simulink model "Sim_LQG_LTR_pheno"  (R2015a)
settings: Solver=ode45  StartTime=0.0  StopTime=t_run  RelTol=1e-3
values from neighbouring files (symbols this model uses):
  Cd = SYSd.c    [LQG_LTR_fen.m]    (also in LQG_LTR_ident.m; LQG_LTR_pheno.m)
  Dd = SYSd.d    [LQG_LTR_fen.m]    (also in LQG_LTR_ident.m; LQG_LTR_pheno.m)
  Gamma = SYSd.b    [LQG_LTR_fen.m]    (also in LQG_LTR_ident.m; LQG_LTR_pheno.m)
  hinicial = [9 7 0 0]    [LQG_LTR_fen.m]    (also in LQG_LTR_ident.m; LQG_LTR_pheno.m; Model.m = [hi1 hi2 0 0])
  Kf = minreal(ss(Kc,'minimal'),1e-4)    [LQG_LTR_fen.m]    (also in LQG_LTR_ident.m; LQG_LTR_pheno.m)
  Phi = SYSd.a    [LQG_LTR_fen.m]    (also in LQG_LTR_ident.m; LQG_LTR_pheno.m)
  Ts = 0.1    [LQG_LTR_fen.m]    (also in LQG_LTR_ident.m; LQG_LTR_pheno.m)
settings Model: Creator=pcosta  LastModifiedBy=lca

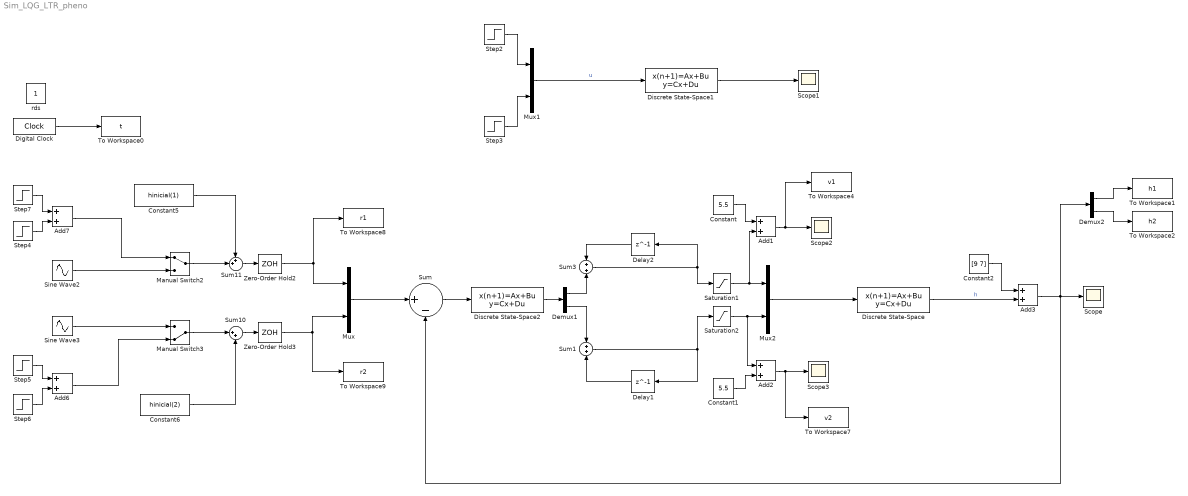
== system Sim_LQG_LTR_pheno ==
  Add{1..3,6..7} (5 alike) : Sum
  Constant : Constant  Value=5.5
  Constant1 : Constant  Value=5.5
  Constant2 : Constant  Value=[9 7]
  Constant5 : Constant  Value=hinicial(1)  SampleTime=Ts
  Constant6 : Constant  Value=hinicial(2)  SampleTime=Ts
  Delay1 : Delay  DelayLength=1  InitialCondition=0  SampleTime=Ts
  Delay2 : Delay  DelayLength=1  InitialCondition=0  SampleTime=Ts
  Demux1 : Demux  Outputs=2
  Demux2 : Demux  Outputs=2
  Digital Clock : DigitalClock  SampleTime=Ts
  Discrete State-Space : DiscreteStateSpace  A=Phi  B=Gamma  C=Cd  D=Dd  SampleTime=Ts
  Discrete State-Space1 : DiscreteStateSpace  A=Phi  B=Gamma  C=Cd  D=Dd  SampleTime=Ts
  Discrete State-Space2 : DiscreteStateSpace  A=Kf.a  B=Kf.b  C=Kf.c  D=Kf.d  SampleTime=Ts
  Manual Switch2 : ManualSwitch
  Manual Switch3 : ManualSwitch  CurrentSetting=0
  Mux : Mux  Inputs=2
  Mux1 : Mux  Inputs=2
  Mux2 : Mux  Inputs=2
  Saturation1 : Saturate  UpperLimit=4.5  LowerLimit=-5.5
  Saturation2 : Saturate  UpperLimit=4.5  LowerLimit=-5.5
  Scope{,1..3} (4 alike) : Scope
      Scope settings: MaxDataPoints=500000
      Scope2 settings: SaveName=ScopeData2  MaxDataPoints=500000
      Scope3 settings: SaveName=ScopeData3
  Sine Wave2 : Sin  Frequency=0.1  SampleTime=0
  Sine Wave3 : Sin  Frequency=0.1  Phase=pi/2  SampleTime=0
  Step2 : Step  Time=0  After=5.5  SampleTime=Ts
  Step3 : Step  Time=0  After=5.5  SampleTime=Ts
  Step4 : Step  Time=400  After=-3  SampleTime=0  ZeroCross=off
  Step5 : Step  Time=200  After=3  SampleTime=0  ZeroCross=off
  Step6 : Step  Time=600  After=-3  SampleTime=0  ZeroCross=off
  Step7 : Step  Time=10  After=3  SampleTime=0  ZeroCross=off
  Sum : Sum  Inputs=|+-
  Sum1 : Sum
  Sum10 : Sum  Inputs=|++
  Sum11 : Sum  Inputs=++|
  Sum3 : Sum
  To Workspace0 : ToWorkspace  VariableName=t  SampleTime=-1
  To Workspace1 : ToWorkspace  VariableName=h1  SampleTime=-1
  To Workspace2 : ToWorkspace  VariableName=h2  SampleTime=-1
  To Workspace4 : ToWorkspace  VariableName=v1  SampleTime=-1
  To Workspace7 : ToWorkspace  VariableName=v2  SampleTime=-1
  To Workspace8 : ToWorkspace  VariableName=r1  SampleTime=-1
  To Workspace9 : ToWorkspace  VariableName=r2  SampleTime=-1
  Zero-Order Hold2 : ZeroOrderHold  SampleTime=Ts
  Zero-Order Hold3 : ZeroOrderHold  SampleTime=Ts
  rds : Constant  IOType=siggen
  wires:
  Mux/1 -> Sum/1
  Discrete State-Space1/1 -> Scope1/1
  Mux1/1 -> Discrete State-Space1/1  "u"
  Step2/1 -> Mux1/1
  Step3/1 -> Mux1/2
  Discrete State-Space2/1 -> Demux1/1
  Sum3/1 -> Saturation1/1, Delay2/1
  Delay2/1 -> Sum3/1
  Sum1/1 -> Saturation2/1, Delay1/1
  Demux1/1 -> Sum3/2
  Saturation2/1 -> Mux2/2, Add2/1
  Saturation1/1 -> Add1/2, Mux2/1
  Constant/1 -> Add1/1
  Add1/1 -> To Workspace4/1, Scope2/1
  Add2/1 -> Scope3/1, To Workspace7/1
  Constant1/1 -> Add2/2
  Constant2/1 -> Add3/1
  Add3/1 -> Sum/2, Demux2/1, Scope/1
  Demux2/1 -> To Workspace1/1
  Demux2/2 -> To Workspace2/1
  Digital Clock/1 -> To Workspace0/1
  Sum/1 -> Discrete State-Space2/1
  Demux1/2 -> Sum1/1
  Delay1/1 -> Sum1/2
  Sum10/1 -> Zero-Order Hold3/1
  Constant6/1 -> Sum10/2
  Step4/1 -> Add7/2
  Step7/1 -> Add7/1
  Constant5/1 -> Sum11/1
  Step5/1 -> Add6/1
  Step6/1 -> Add6/2
  Sum11/1 -> Zero-Order Hold2/1
  Zero-Order Hold2/1 -> Mux/1, To Workspace8/1
  Add7/1 -> Manual Switch2/1
  Sine Wave2/1 -> Manual Switch2/2
  Sine Wave3/1 -> Manual Switch3/1
  Add6/1 -> Manual Switch3/2
  Manual Switch3/1 -> Sum10/1
  Manual Switch2/1 -> Sum11/2
  Zero-Order Hold3/1 -> Mux/2, To Workspace9/1
  Discrete State-Space/1 -> Add3/2  "h"
  Mux2/1 -> Discrete State-Space/1
